simulink model "Likitha_Version_9_2"  (R2025b)
settings: Solver=VariableStepAuto  StartTime=0.0  StopTime=0.3  RelTol=1e-3
undefined symbols (not defined in the file): Ion, Lithium
libraries: spsBatteryLib x50, spsSeriesRLCBranchLib x15, spsCurrentMeasurementLib x10, spsVoltageMeasurementLib x10, spsIdealSwitchLib x9, spsMosfetLib x7, slpidlib x4, spsPWMGeneratorDCDCLib x2, spspowerguiLib x2, spsACVoltageSourceLib x1, eeHysteresisControl x1, spsDCMachineLib x1
(part 4 of 4)

== matlab function Likitha_Version_9_2/Subsystem3/MATLAB Function ==
  settings: updateMethod=DISCRETE
  data: t input; V output; I output; P output; SOC output; T output
function [V, I, P, SOC, T] = HardwareEmulator(t)
% HardwareEmulator - Generates synthetic battery data for testing
% 
% Input:
%   t : current simulation time (s) from a Clock block
%
% Outputs:
%   V   : pack voltage (V)
%   I   : pack current (A) - positive for discharge
%   P   : pack power (W)
%   SOC : state of charge (%)
%   T   : temperature (°C) - constant 25

% -------------------------------------------------------------------------
% Internal parameters (adjust to match your battery pack)
capacity = 50;          % nominal capacity (Ah)
I_nom = 30;             % discharge current (A)
% Linear voltage model: V = a * SOC + b   (at SOC in %)
a = 0.2;                % V/% (voltage change per % SOC)
b = 140;                % V at 0% SOC
T_nom = 25;             % constant temperature (°C)
% -------------------------------------------------------------------------

persistent lastTime lastSOC

% Initialize on first call
if isempty(lastTime)
    lastTime = t;
    lastSOC = 100;      % start fully charged
end

% Time step
dt = t - lastTime;
if dt < 0
    dt = 0;   % protect against negative time (should not happen)
end

% Update SOC using Coulomb counting
% dSOC (%) = (I * dt) / (capacity * 3600) * 100
dSOC = (I_nom * dt) / (capacity * 3600) * 100;
lastSOC = lastSOC - dSOC;   % discharge reduces SOC

% Keep SOC within [0, 100]
lastSOC = max(0, min(100, lastSOC));

% Compute outputs
SOC = lastSOC;
I = I_nom;
V = a * SOC + b;
P = V * I;
T = T_nom;

% Update last time for next step
lastTime = t;

end

== matlab function Likitha_Version_9_2/Subsystem4/MATLAB Function ==
  data: V_meas input; SOC_est output; I_meas input; P_meas input; SOC_ext input; T_meas input; dt input; Vp1_est output; Vp2_est output; R0_est output; Cap_est output; OCV_est output; Vfilt output
function [SOC_est, Vp1_est, Vp2_est, R0_est, Cap_est, OCV_est, Vfilt] = AEKF_Hardware(...
    V_meas, I_meas, P_meas, SOC_ext, T_meas, dt)

% Adaptive Extended Kalman Filter for hardware branch
% All persistent variables declared at top level (required for code generation)

persistent x P Q R R_SOC R0 R1 C1 R2 C2 nominal_capacity
persistent first_run

% -------------------------------------------------------------------------
% Initialize on first call
if isempty(first_run)
    nominal_capacity = 50;      % Ah
    R0 = 0.05;                  % Ohm
    R1 = 0.02;                  % Ohm
    C1 = 2000;                  % Farad
    R2 = 0.03;                  % Ohm
    C2 = 5000;                  % Farad

    % State vector: [SOC(%); Vp1(V); Vp2(V); bias(V); invCap(1/Ah)]
    x = [100; 0; 0; 0; 1/nominal_capacity];
    P = diag([1, 0.1, 0.1, 0.01, 1e-6]);          % initial covariance
    Q = diag([0.01, 0.001, 0.001, 1e-6, 1e-8]);   % process noise
    R = 0.1;                                        % voltage measurement noise
    R_SOC = 1.0;                                    % external SOC measurement noise

    first_run = 1;
end

% -------------------------------------------------------------------------
% Time constants
tau1 = max(R1*C1, 1e-6);
tau2 = max(R2*C2, 1e-6);

% -------------------------------------------------------------------------
% Prediction step (a priori)
SOC = x(1);
Vp1 = x(2);
Vp2 = x(3);
bias = x(4);
invCap = x(5);
Cap = 1 / max(invCap, 1e-6);   % capacity in Ah

alpha1 = exp(-dt / tau1);
alpha2 = exp(-dt / tau2);

x_pred = [SOC - (I_meas * dt) / (3600 * Cap);
          alpha1 * Vp1 + (1 - alpha1) * R1 * I_meas;
          alpha2 * Vp2 + (1 - alpha2) * R2 * I_meas;
          bias;
          invCap];

F = [1, 0, 0, 0,  (I_meas * dt) / (3600 * Cap^2);
     0, alpha1, 0, 0, 0;
     0, 0, alpha2, 0, 0;
     0, 0, 0, 1, 0;
     0, 0, 0, 0, 1];

P_pred = F * P * F' + Q;

% -------------------------------------------------------------------------
% OCV model (simplified linear – replace with lookup if needed)
OCV = 0.04 * SOC + 3.0;          % V
dOCV_dSOC = 0.04;

% -------------------------------------------------------------------------
% Measurement update (voltage + external SOC)
V_pred = OCV - I_meas * R0 - Vp1 - Vp2 + bias;
H = [dOCV_dSOC, -1, -1, 1, 0;    % for voltage
     1,         0,  0,  0, 0];    % for external SOC

z = [V_meas; SOC_ext];
z_pred = [V_pred; SOC];
R_mat = [R, 0; 0, R_SOC];

y = z - z_pred;
S = H * P_pred * H' + R_mat;
K = P_pred * H' / S;

x_upd = x_pred + K * y;
P_upd = (eye(5) - K * H) * P_pred;

% -------------------------------------------------------------------------
% Apply constraints
x_upd(1) = max(0, min(100, x_upd(1)));                       % SOC 0-100%
x_upd(5) = max(1/(2*nominal_capacity), min(1/(0.5*nominal_capacity), x_upd(5)));

x = x_upd;
P = P_upd;

% -------------------------------------------------------------------------
% Outputs
SOC_est = x(1);
Vp1_est = x(2);
Vp2_est = x(3);
bias_est = x(4);
Cap_est = 1 / x(5);
R0_est = R0;                     % could be made adaptive later
OCV_est = OCV;
Vfilt = OCV_est - I_meas * R0 - Vp1_est - Vp2_est + bias_est;

end

== matlab function Likitha_Version_9_2/Subsystem5/MATLAB Function ==
  settings: updateMethod=DISCRETE  sampleTime=0.1
  data: SOC output double size=1; SOH output double size=1; SOP output double size=1; SOC_est input double size=1; DOD output double size=1; ROH output double size=1; Vp1_est input double size=1; Vp2_est input double size=1; R0_est input double size=1; RUL output double size=1; CycleCount output double size=1; V_avg output double size=1; Cap_est input double size=1; OCV_est input double size=1; Vfilt input double size=1; I_meas input double size=1; V_meas input double size=1; T_meas input double size=1; dt input double size=1; timestamp input; I_avg output double size=1; P_avg output double size=1; stress_idx output double size=1; aging_rate_frac output double size=1; energy_kWh output double size=1; degrad_idx output double size=1; T_idx output double size=1; health_idx output double size=1; I_peak output double size=1; V_min output double size=1; T_max output double size=1; Ah_charge_total output double size=1; Ah_discharge_total output double size=1; overtime_sec output double size=1; enableWOA input double size=1
function [SOC, SOH, SOP, DOD, ROH, RUL, CycleCount, ...
          V_avg, I_avg, P_avg, stress_idx, aging_rate_frac, energy_kWh, ...
          degrad_idx, T_idx, health_idx, I_peak, V_min, T_max, ...
          Ah_charge_total, Ah_discharge_total, overtime_sec] = ...
    HybridParameterEstimator_WOA(...
    SOC_est, Vp1_est, Vp2_est, R0_est, Cap_est, OCV_est, Vfilt, ...
    I_meas, V_meas, T_meas, dt, timestamp, enableWOA)

% Hybrid Parameter Estimator with Whale Optimization
% Code‑generation compatible – no tic/toc, all arrays preallocated
%
% Inputs (13 total, all scalar):
%   SOC_est, Vp1_est, Vp2_est, R0_est, Cap_est, OCV_est, Vfilt – from AEKF
%   I_meas, V_meas, T_meas, dt – raw measurements
%   timestamp – current simulation time (from Clock)
%   enableWOA – flag to enable WOA optimization (0 or 1)
%
% Outputs (22 total, all scalar):
%   SOC, SOH, SOP, DOD, ROH, RUL, CycleCount,
%   V_avg, I_avg, P_avg, stress_idx, aging_rate_frac, energy_kWh,
%   degrad_idx, T_idx, health_idx, I_peak, V_min, T_max,
%   Ah_charge_total, Ah_discharge_total, overtime_sec

% -------------------------------------------------------------------------
% Internal constants
nominal_capacity = 50;      % Ah
nominal_resistance = 0.05;  % Ohm
windowSize_avg = 100;       % for moving averages
% -------------------------------------------------------------------------

persistent cycleCount lastSOC V_avg_buf I_avg_buf P_avg_buf bufferIdx
persistent Ah_charge Ah_discharge overtemp_time lastTempTime
persistent E_throughput I_peak_val V_min_val T_max_val
persistent woa_params lastWOATime

% Initialize all persistent variables
if isempty(cycleCount)
    cycleCount = 0;
    lastSOC = SOC_est;
    
    % Buffers for averages
    V_avg_buf = zeros(windowSize_avg, 1);
    I_avg_buf = zeros(windowSize_avg, 1);
    P_avg_buf = zeros(windowSize_avg, 1);
    bufferIdx = 1;
    
    % Accumulators
    Ah_charge = 0;
    Ah_discharge = 0;
    overtemp_time = 0;
    lastTempTime = -inf;      % last time temperature warning was issued
    
    E_throughput = 0;
    I_peak_val = 0;
    V_min_val = inf;
    T_max_val = -inf;
    
    % WOA parameters
    woa_params = struct('R0_opt', R0_est, 'Cap_opt', Cap_est, ...
                        'alpha_opt', 0.1, 'beta_opt', 0.05);
    lastWOATime = -inf;
end

% -------------------------------------------------------------------------
% Update circular buffers for averages
V_avg_buf(bufferIdx) = V_meas;
I_avg_buf(bufferIdx) = I_meas;
P_avg_buf(bufferIdx) = V_meas * I_meas;
bufferIdx = mod(bufferIdx, windowSize_avg) + 1;

V_avg = mean(V_avg_buf);
I_avg = mean(I_avg_buf);
P_avg = mean(P_avg_buf);

% -------------------------------------------------------------------------
% Cycle counting
if lastSOC <= 20 && SOC_est >= 80
    cycleCount = cycleCount + 1;
elseif lastSOC >= 80 && SOC_est <= 20
    cycleCount = cycleCount + 1;
end
lastSOC = SOC_est;
CycleCount = cycleCount;

% -------------------------------------------------------------------------
% Update energy and charge throughput
dAh = abs(I_meas) * dt / 3600;
E_throughput = E_throughput + abs(V_meas * I_meas) * dt / 3600 / 1000;
energy_kWh = E_throughput;

if I_meas < -0.1  % charging
    Ah_charge = Ah_charge + abs(I_meas) * dt / 3600;
elseif I_meas > 0.1  % discharging
    Ah_discharge = Ah_discharge + I_meas * dt / 3600;
end
Ah_charge_total = Ah_charge;
Ah_discharge_total = Ah_discharge;

% -------------------------------------------------------------------------
% Peak tracking with decay
I_peak_val = max(abs(I_meas), 0.999 * I_peak_val);
I_peak = I_peak_val;
V_min_val = min(V_meas, V_min_val + 0.001);
V_min = V_min_val;
T_max_val = max(T_meas, T_max_val - 0.01);
T_max = T_max_val;

% -------------------------------------------------------------------------
% Temperature monitoring
if T_meas > 45
    overtemp_time = overtemp_time + dt;
    if (timestamp - lastTempTime) >= 60
        % Issue warning (simulated)
        lastTempTime = timestamp;
    end
end
overtime_sec = overtemp_time;

% -------------------------------------------------------------------------
% Whale Optimization Algorithm (runs every 300 seconds if enabled)
if enableWOA && (timestamp - lastWOATime) >= 300
    % Use recent data for optimization (simplified features)
    X_train = [V_avg_buf, I_avg_buf, P_avg_buf];
    Y_train = mean(V_avg_buf) * ones(size(X_train,1), 1);  % target

    n_whales = 10;
    n_iter = 20;

    % Initialize whale positions
    whales = zeros(n_whales, 2);
    for i = 1:n_whales
        whales(i,1) = woa_params.R0_opt * (0.8 + 0.4*rand());
        whales(i,2) = woa_params.Cap_opt * (0.9 + 0.2*rand());
    end

    % Preallocate fitness array
    fitness = zeros(n_whales, 1);
    best_whale = whales(1,:);
    best_fit = inf;

    for iter = 1:n_iter
        a = 2 - 2*iter/n_iter;   % linearly decreases from 2 to 0

        % Evaluate fitness for each whale
        for w = 1:n_whales
            R0_test = whales(w,1);
            Cap_test = whales(w,2);
            V_pred = OCV_est - I_meas * R0_test - Vp1_est - Vp2_est;
            err = V_meas - V_pred;
            fitness(w) = err^2;   % mean squared error (simplified)
        end

        % Find best whale
        [min_fit, min_idx] = min(fitness);
        if min_fit < best_fit
            best_fit = min_fit;
            best_whale = whales(min_idx, :);
        end

        % Update positions
        for w = 1:n_whales
            r1 = rand(); r2 = rand();
            A = 2*a*r1 - a;
            C = 2*r2;

            if rand() < 0.5
                if abs(A) < 1
                    % Encircling prey
                    D = abs(C * best_whale - whales(w,:));
                    whales(w,:) = best_whale - A .* D;
                else
                    % Search for prey
                    rand_idx = randi(n_whales);
                    D = abs(C * whales(rand_idx,:) - whales(w,:));
                    whales(w,:) = whales(rand_idx,:) - A .* D;
                end
            else
                % Bubble-net attacking (spiral)
                D = abs(best_whale - whales(w,:));
                L = -1 + 2*rand();
                whales(w,:) = D .* exp(1)^(L) .* cos(2*pi*L) + best_whale;
            end

            % Constrain to reasonable ranges
            whales(w,1) = max(0.01, min(0.1, whales(w,1)));
            whales(w,2) = max(40,   min(60,   whales(w,2)));
        end
    end

    % Update optimized parameters
    woa_params.R0_opt = best_whale(1);
    woa_params.Cap_opt = best_whale(2);

    lastWOATime = timestamp;
end

% -------------------------------------------------------------------------
% Use optimized parameters if WOA has run at least once
if enableWOA && lastWOATime > -inf
    R0_adaptive = woa_params.R0_opt;
    Cap_adaptive = woa_params.Cap_opt;
else
    R0_adaptive = R0_est;
    Cap_adaptive = Cap_est;
end

% -------------------------------------------------------------------------
% Basic parameters
SOC = SOC_est;
SOH = (Cap_adaptive / nominal_capacity) * 100;
SOH = max(0, min(100, SOH));

DOD = 100 - SOC;
ROH = R0_adaptive;

% State of Power (SOP)
OCV_simple = 0.04 * SOC + 3.0;
Vmin = 2.7;
I_max_dis = (OCV_simple - Vmin) / (ROH + 1e-6);
SOP = I_max_dis * Vmin;

% -------------------------------------------------------------------------
% Stress Index
C_rate = abs(I_meas) / Cap_adaptive;
thermal_stress = (T_meas - 25)^2 / 625;
electrical_stress = (C_rate / 3)^2;
stress_idx = min(1, 0.6 * electrical_stress + 0.4 * thermal_stress);

% -------------------------------------------------------------------------
% Aging rate and RUL
if cycleCount > 0
    base_aging = (100 - SOH) / cycleCount;
    T_accel = exp(0.05 * (T_meas - 25));
    C_accel = 1 + 0.2 * (C_rate - 0.5);
    C_accel = max(1, min(2, C_accel));
    aging_rate_per_cycle = base_aging * T_accel * C_accel;
else
    aging_rate_per_cycle = 0.01;
end
aging_rate_frac = aging_rate_per_cycle / 100;

if SOH > 80
    cycles_to_80 = (SOH - 80) / aging_rate_per_cycle;
    RUL = max(0, cycles_to_80);
else
    RUL = 0;
end

% -------------------------------------------------------------------------
% Degradation and health indices
degrad_idx = 1 - SOH/100;
T_idx = max(0, min(1, 1 - abs(T_meas - 25)/50));
health_idx = 0.5*(SOH/100) + 0.3*(1-stress_idx) + 0.2*T_idx;

% -------------------------------------------------------------------------
% Ensure all outputs are real
vars = {SOC, SOH, SOP, DOD, ROH, RUL, CycleCount, V_avg, I_avg, P_avg, ...
        stress_idx, aging_rate_frac, energy_kWh, degrad_idx, T_idx, ...
        health_idx, I_peak, V_min, T_max, Ah_charge_total, ...
        Ah_discharge_total, overtime_sec};
for i = 1:length(vars)
    if ~isreal(vars{i})
        vars{i} = real(vars{i});
    end
end

% Unpack outputs (this is just for clarity)
[SOC, SOH, SOP, DOD, ROH, RUL, CycleCount, V_avg, I_avg, P_avg, ...
 stress_idx, aging_rate_frac, energy_kWh, degrad_idx, T_idx, ...
 health_idx, I_peak, V_min, T_max, Ah_charge_total, ...
 Ah_discharge_total, overtime_sec] = vars{:};

end

== matlab function Likitha_Version_9_2/Subsystem5/MATLAB Function1 ==
  settings: updateMethod=DISCRETE
  data: SOC input double size=1; SOH input double size=1; SOP input double size=1; DOD input double size=1; ROH input double size=1; RUL input double size=1; CycleCount input double size=1; V_avg input double size=1; I_avg input double size=1; P_avg input double size=1; stress_idx input double size=1; aging_rate_frac input double size=1; energy_kWh input double size=1; degrad_idx input double size=1; T_idx input double size=1; health_idx input double size=1; I_peak input double size=1; V_min input double size=1; T_max input double size=1; Ah_charge_total input double size=1; Ah_discharge_total input double size=1; overtime_sec input double size=1; timestamp input double size=1; windowSize input double size=1; stepSize input double size=1; enableGPR input double size=1; features output double size=[1 396]; labels output double size=[1 2]; newDataReady output double size=1; anomalyScores output double size=[1 2]
function [features, labels, newDataReady, anomalyScores] = ...
    MultiScaleFeatureEngineer(...
    SOC, SOH, SOP, DOD, ROH, RUL, CycleCount, ...
    V_avg, I_avg, P_avg, stress_idx, aging_rate_frac, energy_kWh, ...
    degrad_idx, T_idx, health_idx, I_peak, V_min, T_max, ...
    Ah_charge_total, Ah_discharge_total, overtime_sec, ...
    timestamp, windowSize, stepSize, enableGPR)

% Multi‑Scale Feature Engineer – fixed‑size outputs
% Inputs: 22 parameters + timestamp, windowSize, stepSize, enableGPR (all scalar)
% Outputs: features [1x396], labels [1x2], newDataReady (scalar), anomalyScores [1x2]

% -------------------------------------------------------------------------
% Internal constants
maxSamples = 2000;          % size of raw data circular buffer
n_scales = 3;                % number of downsampling scales
featureLen = 22 * n_scales * 6;   % 22 × 3 × 6 = 396
% -------------------------------------------------------------------------

persistent buffer timeBuffer bufferIdx counter lastOutputTime
persistent gprEnabled trainedGPR

% Initialize persistent variables
if isempty(buffer)
    buffer = zeros(maxSamples, 22);
    timeBuffer = zeros(maxSamples, 1);
    bufferIdx = 1;
    counter = 0;
    lastOutputTime = -inf;
    gprEnabled = (enableGPR ~= 0);   % convert to logical
    trainedGPR = false;
end

% Current feature vector (1×22)
currentFeatures = [SOC, SOH, SOP, DOD, ROH, RUL, CycleCount, ...
                   V_avg, I_avg, P_avg, stress_idx, aging_rate_frac, energy_kWh, ...
                   degrad_idx, T_idx, health_idx, I_peak, V_min, T_max, ...
                   Ah_charge_total, Ah_discharge_total, overtime_sec];

% Store in circular buffer
buffer(bufferIdx, :) = currentFeatures;
timeBuffer(bufferIdx) = timestamp;
bufferIdx = mod(bufferIdx, maxSamples) + 1;
counter = counter + 1;

% Default outputs
features = zeros(1, featureLen);
labels = [0, 0];
newDataReady = 0;
anomalyScores = [0, 0];

% Check if we have enough data to form a window
if counter >= windowSize && (timestamp - lastOutputTime) >= stepSize

    % Extract the most recent window (chronological order)
    if bufferIdx > windowSize
        winIndices = (bufferIdx - windowSize) : (bufferIdx - 1);
    else
        % Wrap around circular buffer
        winIndices = [(maxSamples - windowSize + bufferIdx + 1) : maxSamples, 1:(bufferIdx - 1)];
    end
    windowData = buffer(winIndices, :);

    % -----------------------------------------------------------------
    % Multi‑Scale Feature Extraction
    % -----------------------------------------------------------------
    % Pre‑allocate featVec with zeros to ensure fixed length
    featVec = zeros(1, featureLen);
    pos = 1;
    for scale = 1:n_scales
        ds = windowData(1:scale:end, :);
        if size(ds, 1) < 2
            continue;
        end
        for p = 1:22
            col = ds(:, p);
            % Compute statistics (ensure no NaN)
            m = mean(col);
            s = std(col);
            if s < 1e-6, s = 0; end
            mn = min(col);
            mx = max(col);
            tr = col(end) - col(1);
            ch = sum(abs(diff(col)) > 0.01 * s);
            % Assign to featVec at correct positions
            if pos + 5 <= featureLen
                featVec(pos:pos+5) = [m, s, mn, mx, tr, ch];
                pos = pos + 6;
            end
        end
    end
    % featVec already has zeros beyond pos, so it's always featureLen long.
    features = featVec;

    % Labels = last sample's SOC and SOH
    labels = windowData(end, 1:2);
    newDataReady = 1;

    % Simple GPR anomaly detection (placeholder)
    if gprEnabled && ~trainedGPR && counter > 5 * windowSize
        trainedGPR = true;
    end
    if trainedGPR
        anomalyScores = [var(windowData(:)), std(windowData(:))];
    end

    lastOutputTime = timestamp;
end

end

== matlab function Likitha_Version_9_2/Subsystem5/MATLAB Function2 ==
  data: features input double size=[1 396]; labels input double size=[1 2]; newDataReady input double size=1; SOC_pred output double size=1; algorithmChoice input double size=1; SOH_pred output double size=1; RUL_pred output double size=1; confidence output double size=[1 2]; algoCode output double size=1; metrics output double size=[1 4]; mode input double size=1; earlyStopPercent input double size=1
function [SOC_pred, SOH_pred, RUL_pred, confidence, algoCode, metrics] = ...
    BatteryGPT_Estimator(features, labels, newDataReady, algorithmChoice, mode, earlyStopPercent)

% BatteryGPT Estimator – stores its own training data, fixed‑size
% Inputs:
%   features   : [1x396] feature vector from Block 16
%   labels     : [1x2] actual [SOC, SOH] for this window
%   newDataReady : scalar (1 when new window available)
%   algorithmChoice : scalar (not used)
%   mode       : scalar (1=train, 0=predict)
%   earlyStopPercent : scalar (not used)
%
% Outputs:
%   SOC_pred, SOH_pred, RUL_pred : scalars
%   confidence : [1x2] [conf_SOC, conf_SOH]
%   algoCode   : scalar (algorithm used)
%   metrics    : [1x4] [RMSE_SOC, RMSE_SOH, MAE_SOC, MAE_SOH]

% -------------------------------------------------------------------------
% Internal constants
maxWindows = 200;               % maximum number of windows to store
featureDim = 396;                % feature dimension
% -------------------------------------------------------------------------

persistent featureBuffer labelBuffer windowCount
persistent trainedModel          % will be a struct, initially empty

if isempty(featureBuffer)
    featureBuffer = zeros(maxWindows, featureDim);
    labelBuffer = zeros(maxWindows, 2);
    windowCount = 0;
    % Initialize trainedModel as an empty struct with default fields
    trainedModel = struct('theta_soc', zeros(featureDim+1,1), ...
                          'theta_soh', zeros(featureDim+1,1));
end

% If new data arrives, store it (if we have space)
if newDataReady && windowCount < maxWindows
    windowCount = windowCount + 1;
    featureBuffer(windowCount, :) = features;
    labelBuffer(windowCount, :) = labels;
end

% Default outputs
SOC_pred = labels(1);
SOH_pred = labels(2);
RUL_pred = 0;
confidence = [0.5, 0.5];
algoCode = algorithmChoice;
metrics = zeros(1, 4);

% Train if in training mode and enough data
if mode == 1 && windowCount >= 30
    % Use all stored windows for training
    X = featureBuffer(1:windowCount, :);
    Y = labelBuffer(1:windowCount, :);
    
    % Add bias term
    X_aug = [ones(windowCount, 1), X];   % size windowCount × (featureDim+1)
    
    % Linear regression (placeholder – replace with actual GPT training)
    theta_soc = (X_aug' * X_aug) \ (X_aug' * Y(:, 1));
    theta_soh = (X_aug' * X_aug) \ (X_aug' * Y(:, 2));
    
    % Store model
    trainedModel.theta_soc = theta_soc;
    trainedModel.theta_soh = theta_soh;
    
    % Compute metrics on training data
    Y_pred_soc = X_aug * theta_soc;
    Y_pred_soh = X_aug * theta_soh;
    rmse_soc = sqrt(mean((Y(:,1) - Y_pred_soc).^2));
    rmse_soh = sqrt(mean((Y(:,2) - Y_pred_soh).^2));
    mae_soc  = mean(abs(Y(:,1) - Y_pred_soc));
    mae_soh  = mean(abs(Y(:,2) - Y_pred_soh));
    metrics = [rmse_soc, rmse_soh, mae_soc, mae_soh];
end

% Predict using the latest model (if available)
if isfield(trainedModel, 'theta_soc') && any(trainedModel.theta_soc ~= 0)
    X_curr = [1, features];   % add bias
    SOC_pred = X_curr * trainedModel.theta_soc;
    SOH_pred = X_curr * trainedModel.theta_soh;
    confidence = [0.9, 0.9];
else
    % No model yet – use current labels as fallback
    SOC_pred = labels(1);
    SOH_pred = labels(2);
    confidence = [0.7, 0.7];
end

% Clamp predictions to valid range
SOC_pred = max(0, min(100, SOC_pred));
SOH_pred = max(0, min(100, SOH_pred));

% Estimate RUL from SOH (simple linear model)
if SOH_pred > 80
    RUL_pred = (SOH_pred - 80) / 0.1;   % assume 0.1% loss per cycle
else
    RUL_pred = 0;
end
RUL_pred = max(0, RUL_pred);

end

== matlab function Likitha_Version_9_2/Subsystem5/MATLAB Function3 ==
  data: SOC input double size=1; SOC_pred output double size=1; SOH input double size=1; SOP input double size=1; DOD input double size=1; ROH input double size=1; RUL input double size=1; CycleCount input double size=1; V_avg input double size=1; I_avg input double size=1; P_avg input double size=1; stress_idx input double size=1; aging_rate_frac input double size=1; energy_kWh input double size=1; degrad_idx input double size=1; T_idx input double size=1; health_idx input double size=1; I_peak input double size=1; V_min input double size=1; T_max input double size=1; Ah_charge_total input double size=1; Ah_discharge_total input double size=1; overtime_sec input double size=1; timestamp input double size=1; enableTraining input double size=1; algorithmChoice input double size=1; cloudSync input double size=1; SOH_pred output double size=1; RUL_pred output double size=1; conf_SOC output double size=1; conf_SOH output double size=1; modelTypeCode output double size=1; ensembleWeights output double size=[1 5]
function [SOC_pred, SOH_pred, RUL_pred, conf_SOC, conf_SOH, modelTypeCode, ensembleWeights] = ...
    FederatedEnsemblePredictor(...
    SOC, SOH, SOP, DOD, ROH, RUL, CycleCount, ...
    V_avg, I_avg, P_avg, stress_idx, aging_rate_frac, energy_kWh, ...
    degrad_idx, T_idx, health_idx, I_peak, V_min, T_max, ...
    Ah_charge_total, Ah_discharge_total, overtime_sec, ...
    timestamp, enableTraining, algorithmChoice, cloudSync)

% Federated Ensemble Predictor – fully fixed‑size, code‑generation ready
% All persistent arrays have fixed dimensions, no tic/toc, no strings.
%
% Inputs (26 total, all scalar):
%   22 battery parameters (from SOC to overtime_sec)
%   timestamp       : current simulation time
%   enableTraining  : 1 to enable online learning
%   algorithmChoice : (reserved) not used
%   cloudSync       : (reserved) not used
%
% Outputs:
%   SOC_pred, SOH_pred, RUL_pred, conf_SOC, conf_SOH : scalars
%   modelTypeCode                : scalar (1 = ensemble)
%   ensembleWeights              : [1×5] vector of ensemble member weights

% -------------------------------------------------------------------------
% Internal constants
n_models = 5;               % number of ensemble members
maxBuffer = 200;            % max samples to store for training
featureDim = 22;            % number of input features
% -------------------------------------------------------------------------

persistent X_buffer Y_buffer bufferIdx sampleCount
persistent model_weights ensemble_models lastTrainTime
persistent prediction_history histIdx

% Initialize persistent variables with fixed sizes
if isempty(X_buffer)
    X_buffer = zeros(maxBuffer, featureDim);
    Y_buffer = zeros(maxBuffer, 2);
    bufferIdx = 1;
    sampleCount = 0;

    % Ensemble weights (equal initially)
    model_weights = ones(1, n_models) / n_models;

    % Pre‑allocate ensemble models as a struct array using repmat
    % Each model has fields: w (weights, [22×1]), b (scalar), unc (scalar)
    emptyModel = struct('w', zeros(featureDim,1), 'b', 0, 'unc', 0.1);
    ensemble_models = repmat(emptyModel, n_models, 1);

    lastTrainTime = -inf;

    % Circular buffer for prediction history (for uncertainty calibration)
    prediction_history.soc = zeros(1, 100);
    prediction_history.soh = zeros(1, 100);
    prediction_history.actual_soc = zeros(1, 100);
    prediction_history.actual_soh = zeros(1, 100);
    histIdx = 1;
end

% Current feature vector (1×22)
X_curr = [SOC, SOH, SOP, DOD, ROH, RUL, CycleCount, ...
          V_avg, I_avg, P_avg, stress_idx, aging_rate_frac, energy_kWh, ...
          degrad_idx, T_idx, health_idx, I_peak, V_min, T_max, ...
          Ah_charge_total, Ah_discharge_total, overtime_sec];

% Store sample in buffer if training enabled
if enableTraining && timestamp > 0
    X_buffer(bufferIdx, :) = X_curr;
    Y_buffer(bufferIdx, :) = [SOC, SOH];
    bufferIdx = mod(bufferIdx, maxBuffer) + 1;
    if sampleCount < maxBuffer
        sampleCount = sampleCount + 1;
    end
end

% -------------------------------------------------------------------------
% Ensemble prediction
% -------------------------------------------------------------------------
ensemble_pred_soc = zeros(1, n_models);
ensemble_pred_soh = zeros(1, n_models);

for i = 1:n_models
    % Linear model: y = X * w + b
    ensemble_pred_soc(i) = X_curr * ensemble_models(i).w + ensemble_models(i).b;
    ensemble_pred_soh(i) = X_curr * ensemble_models(i).w + ensemble_models(i).b; % same for simplicity
end

% Weighted ensemble prediction
SOC_pred = model_weights * ensemble_pred_soc';
SOH_pred = model_weights * ensemble_pred_soh';

% -------------------------------------------------------------------------
% Uncertainty estimation
% -------------------------------------------------------------------------
% Aleatoric: average model uncertainty
aleatoric = mean([ensemble_models.unc]);

% Epistemic: standard deviation of predictions
epistemic = (std(ensemble_pred_soc) + std(ensemble_pred_soh)) / 2;

% Confidence (inverse of uncertainty)
conf_SOC = 1 - tanh(aleatoric + epistemic);
conf_SOH = conf_SOC;

% -------------------------------------------------------------------------
% Online learning (retrain every 300 seconds if enough samples)
% -------------------------------------------------------------------------
if enableTraining && sampleCount >= 50 && (timestamp - lastTrainTime) >= 300
    % Use all stored samples
    X = X_buffer(1:sampleCount, :);
    Y = Y_buffer(1:sampleCount, :);

    % Retrain each ensemble member on a different bootstrap sample
    for i = 1:n_models
        % Bootstrap sampling
        idx = randi(sampleCount, sampleCount, 1);
        Xb = X(idx, :);
        Yb = Y(idx, :);

        % Simple linear regression: theta = (X'*X)\X'*Y
        Xb_aug = [ones(sampleCount,1), Xb];                % size sampleCount × (featureDim+1)
        theta_soc = (Xb_aug' * Xb_aug) \ (Xb_aug' * Yb(:,1));  % (featureDim+1) × 1
        theta_soh = (Xb_aug' * Xb_aug) \ (Xb_aug' * Yb(:,2));

        % Update model weights – use explicit indices for fixed size
        ensemble_models(i).w = theta_soc(2:featureDim+1);   % features weights, 22×1
        ensemble_models(i).b = theta_soc(1);                % bias

        % Estimate uncertainty from residual
        Y_pred = Xb_aug * theta_soc;
        ensemble_models(i).unc = mean(abs(Yb(:,1) - Y_pred));
    end

    % Update ensemble weights based on recent performance (inverse uncertainty)
    unc_vals = zeros(1, n_models);
    for i = 1:n_models
        unc_vals(i) = ensemble_models(i).unc;
    end
    inv_unc = 1 ./ (unc_vals + 1e-6);
    model_weights = inv_unc / sum(inv_unc);

    lastTrainTime = timestamp;
end

% -------------------------------------------------------------------------
% Update prediction history for calibration (simplified)
% -------------------------------------------------------------------------
prediction_history.soc(histIdx) = SOC_pred;
prediction_history.soh(histIdx) = SOH_pred;
prediction_history.actual_soc(histIdx) = SOC;
prediction_history.actual_soh(histIdx) = SOH;
histIdx = mod(histIdx, 100) + 1;

% -------------------------------------------------------------------------
% RUL estimation (simple)
% -------------------------------------------------------------------------
if SOH_pred > 80
    RUL_pred = (SOH_pred - 80) / 0.1;
else
    RUL_pred = 0;
end
RUL_pred = max(0, RUL_pred);

% Clamp outputs
SOC_pred = max(0, min(100, SOC_pred));
SOH_pred = max(0, min(100, SOH_pred));

% Model type code (1 = ensemble) – must be double, not string
modelTypeCode = 1;

% Ensemble weights output (fixed 1×5)
ensembleWeights = model_weights;

end

== matlab function Likitha_Version_9_2/Subsystem6/MATLAB Function ==
  settings: updateMethod=DISCRETE
  data: sim_params input double size=[1 22]; V_dif output double size=1; hw_params input double size=[1 22]; timestamp input double size=1; sim_algo input double size=1; hw_algo input double size=1; reset input double size=1; I_dif output double size=1; P_dif output double size=1; SOC_dif output double size=1; SCH_dif output double size=1; mse_V output double size=1; mse_I output double size=1; mse_SOC output double size=1; mse_SCH output double size=1; max_cell_imbalance_sim output double size=1; max_cell_imbalance_hv output double size=1; charging_efficiency output double size=1; discharging_efficiency output double size=1; coulombic_efficiency output double size=1; slg2_sim output double size=1; algo_hv output double size=1; log_data output double size=[1 66]
function [V_dif, I_dif, P_dif, SOC_dif, SCH_dif, ...
          mse_V, mse_I, mse_SOC, mse_SCH, ...
          max_cell_imbalance_sim, max_cell_imbalance_hv, ...
          charging_efficiency, discharging_efficiency, coulombic_efficiency, ...
          slg2_sim, algo_hv, log_data] = ...
    CompareModules_Final(sim_params, hw_params, timestamp, sim_algo, hw_algo, reset)

% Comparison Block – fixed‑size persistent arrays, code‑generation ready
% Inputs:
%   sim_params : [1x22] vector from simulation branch
%   hw_params  : [1x22] vector from hardware branch
%   timestamp  : current simulation time (scalar)
%   sim_algo   : algorithm code for simulation (scalar)
%   hw_algo    : algorithm code for hardware (scalar)
%   reset      : set to 1 to reset accumulated errors (scalar)
%
% Outputs (17 total):
%   V_dif, I_dif, P_dif, SOC_dif, SCH_dif : instantaneous differences
%   mse_V, mse_I, mse_SOC, mse_SCH        : running RMSE
%   max_cell_imbalance_sim, max_cell_imbalance_hv : cell voltage spreads
%   charging_efficiency, discharging_efficiency, coulombic_efficiency
%   slg2_sim, algo_hv                      : algorithm codes
%   log_data                                : [1x66] vector for CSV logging

% -------------------------------------------------------------------------
% Parameter index mapping (1‑based) – MUST match your upstream blocks
% 1:SOC, 2:SOH, 3:SOP, 4:DOD, 5:ROH, 6:RUL, 7:CycleCount,
% 8:V_avg, 9:I_avg, 10:P_avg, 11:stress_idx, 12:aging_rate_frac, 13:energy_kWh,
% 14:degrad_idx, 15:T_idx, 16:health_idx, 17:I_peak, 18:V_min, 19:T_max,
% 20:Ah_charge_total, 21:Ah_discharge_total, 22:overtime_sec
% -------------------------------------------------------------------------

% Extract simulation parameters
SOC_sim   = sim_params(1);
SOH_sim   = sim_params(2);
RUL_sim   = sim_params(6);
Cycle_sim = sim_params(7);
V_sim     = sim_params(8);
I_sim     = sim_params(9);
P_sim     = sim_params(10);
stress_sim = sim_params(11);
health_sim = sim_params(16);
V_min_sim  = sim_params(18);
V_max_sim  = sim_params(17);   % using I_peak as proxy for max voltage
T_sim      = sim_params(19);   % T_max as temperature proxy
energy_sim = sim_params(13);
charge_sim = sim_params(20) + sim_params(21); % total Ah throughput

% Extract hardware parameters (same indices)
SOC_hw   = hw_params(1);
SOH_hw   = hw_params(2);
RUL_hw   = hw_params(6);
Cycle_hw = hw_params(7);
V_hw     = hw_params(8);
I_hw     = hw_params(9);
P_hw     = hw_params(10);
stress_hw = hw_params(11);
health_hw = hw_params(16);
V_min_hw  = hw_params(18);
V_max_hw  = hw_params(17);
T_hw      = hw_params(19);
energy_hw = hw_params(13);
charge_hw = hw_params(20) + hw_params(21);

% Compute instantaneous differences
V_dif   = V_sim - V_hw;
I_dif   = I_sim - I_hw;
P_dif   = P_sim - P_hw;
SOC_dif = SOC_sim - SOC_hw;
SCH_dif = SOH_sim - SOH_hw;
T_dif   = T_sim - T_hw;          % for logging only
Cycle_dif = Cycle_sim - Cycle_hw;
RUL_dif   = RUL_sim - RUL_hw;
health_dif = health_sim - health_hw;
stress_dif = stress_sim - stress_hw;

% -------------------------------------------------------------------------
% Persistent variables for RMSE (fixed‑size circular buffer)
persistent err_V err_I err_SOC err_SOH err_idx max_errors
persistent cum_energy_sim cum_energy_hw cum_charge_sim cum_charge_hw

% Initialize on first call
if isempty(err_V)
    max_errors = 10000;                        % store up to 10000 samples
    err_V = zeros(1, max_errors);
    err_I = zeros(1, max_errors);
    err_SOC = zeros(1, max_errors);
    err_SOH = zeros(1, max_errors);
    err_idx = 0;
    cum_energy_sim = 0;
    cum_energy_hw  = 0;
    cum_charge_sim = 0;
    cum_charge_hw  = 0;
elseif reset
    % Reinitialize when reset is triggered
    err_V(:) = 0;
    err_I(:) = 0;
    err_SOC(:) = 0;
    err_SOH(:) = 0;
    err_idx = 0;
    cum_energy_sim = 0;
    cum_energy_hw  = 0;
    cum_charge_sim = 0;
    cum_charge_hw  = 0;
end

% Update cumulative values with latest parameters (these are just copies)
cum_energy_sim = energy_sim;
cum_energy_hw  = energy_hw;
cum_charge_sim = charge_sim;
cum_charge_hw  = charge_hw;

% Store errors only when timestamp advances (and not reset)
if timestamp > 0 && ~reset
    err_idx = err_idx + 1;
    if err_idx > max_errors
        % Circular buffer: discard oldest, keep most recent
        err_V(1:end-1) = err_V(2:end);
        err_I(1:end-1) = err_I(2:end);
        err_SOC(1:end-1) = err_SOC(2:end);
        err_SOH(1:end-1) = err_SOH(2:end);
        err_idx = max_errors;
    end
    err_V(err_idx) = V_dif;
    err_I(err_idx) = I_dif;
    err_SOC(err_idx) = SOC_dif;
    err_SOH(err_idx) = SCH_dif;
end

% Compute RMSE from all stored errors
if err_idx > 0
    mse_V   = sqrt(mean(err_V(1:err_idx).^2));
    mse_I   = sqrt(mean(err_I(1:err_idx).^2));
    mse_SOC = sqrt(mean(err_SOC(1:err_idx).^2));
    mse_SCH = sqrt(mean(err_SOH(1:err_idx).^2));
else
    mse_V = 0; mse_I = 0; mse_SOC = 0; mse_SCH = 0;
end

% Cell imbalance (using min and max as proxy)
max_cell_imbalance_sim = V_max_sim - V_min_sim;
max_cell_imbalance_hv  = V_max_hw  - V_min_hw;

% Efficiencies (prevent division by zero)
if cum_energy_hw > 0
    charging_efficiency = cum_energy_sim / cum_energy_hw;
else
    charging_efficiency = 1;
end
if cum_charge_hw > 0
    coulombic_efficiency = cum_charge_sim / cum_charge_hw;
else
    coulombic_efficiency = 1;
end
discharging_efficiency = charging_efficiency; % simplified

% Algorithm codes
slg2_sim = sim_algo;
algo_hv  = hw_algo;

% -------------------------------------------------------------------------
% Build log_data vector – fixed length 1x66
% Order:
%   1 timestamp
%   2-23 sim_params (22)
%   24-45 hw_params (22)
%   46 V_dif, 47 I_dif, 48 P_dif, 49 SOC_dif, 50 SCH_dif,
%   51 T_dif, 52 Cycle_dif, 53 RUL_dif, 54 health_dif, 55 stress_dif
%   56 mse_V, 57 mse_I, 58 mse_SOC, 59 mse_SCH
%   60 max_cell_imbalance_sim, 61 max_cell_imbalance_hv
%   62 charging_efficiency, 63 discharging_efficiency, 64 coulombic_efficiency
%   65 sim_algo, 66 hw_algo
% -------------------------------------------------------------------------
log_data = [timestamp, ...
            sim_params, ...
            hw_params, ...
            V_dif, I_dif, P_dif, SOC_dif, SCH_dif, T_dif, Cycle_dif, RUL_dif, health_dif, stress_dif, ...
            mse_V, mse_I, mse_SOC, mse_SCH, ...
            max_cell_imbalance_sim, max_cell_imbalance_hv, ...
            charging_efficiency, discharging_efficiency, coulombic_efficiency, ...
            sim_algo, hw_algo];

end

== matlab function Likitha_Version_9_2/Controller/BMS ==
  settings: updateMethod=DISCRETE
  data: SOC input; C output; t input
function C = fcn_charge_discharge_time(SOC, t)
% C = 1 → Charge
% C = 0 → Discharge

%% USER SETTINGS
T_charge    = 100;   % Charge duration (sec)
T_discharge = 100;   % Discharge duration (sec)
MaxCycles   = 5;     % Number of cycles

%% Persistent variables
persistent last_value t_ref cycle mode
% mode: 1 = charge, 0 = discharge

if isempty(last_value)
    last_value = 1;      % Start with charging
    t_ref = t;
    cycle = 0;
    mode = 1;
end

%% Stop switching after max cycles
if cycle >= MaxCycles
    C = last_value;
    return;
end

%% Time-based switching
if mode == 1   % Charging
    if (t - t_ref) >= T_charge || SOC >= 80
        mode = 0;       % Switch to discharge
        t_ref = t;
    end
else           % Discharging
    if (t - t_ref) >= T_discharge || SOC <= 20
        mode = 1;       % Switch to charge
        t_ref = t;
        cycle = cycle + 1;  % Count full cycle
    end
end

%% Output
C = mode;
last_value = C;

end

== matlab function Likitha_Version_9_2/Subsystem11/Subsystem/MATLAB Function ==
  data: inputValue input; output output
function output = divideByFifty(inputValue)
% This function divides the input decimal value by 50

output = inputValue / 50;

end

== stateflow chart Likitha_Version_9_2/Charger/5SCCC ==
  state Initialize
    entry:
    signal=1;
    Iref=1*C;
  state fifth_stage
    entry:
    Iref=0.01*C;
  state end
    entry:
    signal=2;
  state back_to_charge
    entry:
    signal=1;
    Iref=0;
  state first_stage
    entry:
    Iref=0.32*C;
  state fourth_stage
    entry:
    Iref=0.057*C;
  state second_stage
    entry:
    Iref=0.1*C;
  state third_stage
    entry:
    Iref=0.1*C;
  back_to_charge -> (junction 27)
  (junction 27) -> end [order 2]
  (default) -> (junction 27)
  Initialize -> (junction 27) [order 2] : [sw==0]
  (junction 27) -> Initialize [order 1] : [sw==1]
  end -> back_to_charge : [sw==1]
  fifth_stage -> end [order 1] : [Vpeak<=Vb]
  first_stage -> Initialize [order 2] : [sw==0]
  fifth_stage -> fourth_stage [order 2] : [sw==0]
  Initialize -> first_stage [order 1] : [Vpeak<=Vb]
  fourth_stage -> fifth_stage [order 1] : [Vpeak<=Vb]
  fourth_stage -> third_stage [order 2] : [sw==0]
  second_stage -> first_stage [order 2] : [sw==0]
  first_stage -> second_stage [order 1] : [Vpeak<=Vb]
  third_stage -> fourth_stage [order 1] : [Vpeak<=Vb]
  second_stage -> third_stage [order 1] : [Vpeak<=Vb]
  third_stage -> second_stage [order 2] : [sw==0]
  data: Vpeak input; Vb input; Iref output; signal output; C input; sw input
